simulink model "Seguidor_Controlador_PI"  (R2016a)
settings: Solver=VariableStepAuto  StartTime=0.0  StopTime=10.0  RelTol=1e-3
undefined symbols (not defined in the file or in its folder): A, B, C, Ki, Kp
settings Model: Creator=Daniel  LastModifiedBy=Daniel

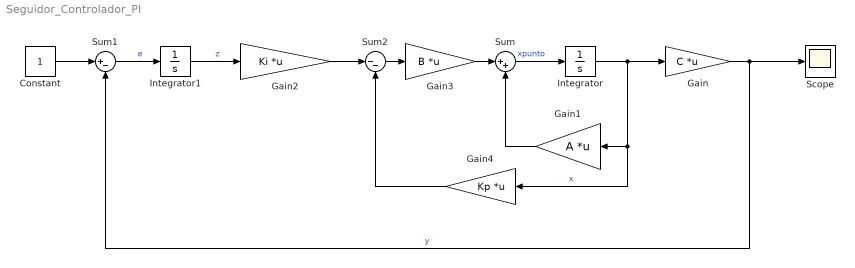
== system Seguidor_Controlador_PI ==
  Constant : Constant
  Gain : Gain  Gain=C  Multiplication=Matrix(K*u) (u vector)
  Gain1 : Gain  Gain=A  Multiplication=Matrix(K*u) (u vector)
  Gain2 : Gain  Gain=Ki  Multiplication=Matrix(K*u) (u vector)
  Gain3 : Gain  Gain=B  Multiplication=Matrix(K*u) (u vector)
  Gain4 : Gain  Gain=Kp  Multiplication=Matrix(K*u) (u vector)
  Integrator : Integrator
  Integrator1 : Integrator
  Scope : Scope
  Sum : Sum  Inputs=|++
  Sum1 : Sum  Inputs=|+-
  Sum2 : Sum  Inputs=|--
  wires:
  Integrator/1 -> Gain4/1, Gain1/1, Gain/1  "x"
  Sum/1 -> Integrator/1  "xpunto"
  Gain1/1 -> Sum/2
  Integrator1/1 -> Gain2/1  "z"
  Sum1/1 -> Integrator1/1  "e"
  Gain/1 -> Scope/1, Sum1/2  "y"
  Constant/1 -> Sum1/1
  Gain2/1 -> Sum2/1
  Sum2/1 -> Gain3/1
  Gain3/1 -> Sum/1
  Gain4/1 -> Sum2/2
